simulink library "findDotPositions_ul"  (R2018b)
settings: Solver=VariableStepAuto  StartTime=0.0  StopTime=10.0  RelTol=1e-3
settings Model: Creator=MAE-NCSUCORE  LastModifiedBy=MAE-NCSUCORE

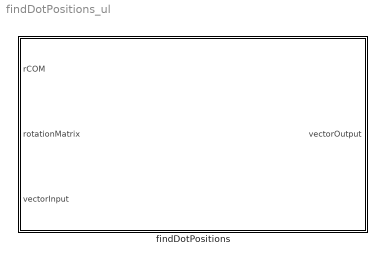
== system findDotPositions_ul ==
  findDotPositions : Subsystem

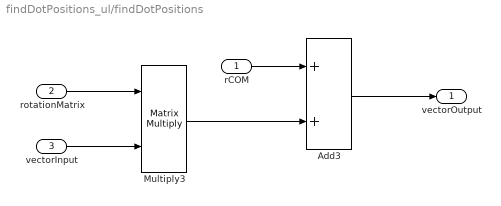
== system findDotPositions_ul/findDotPositions ==
  rCOM : Inport
  rotationMatrix : Inport  Port=2
  vectorInput : Inport  Port=3
  Add3 : Sum
  Multiply3 : Product  Multiplication=Matrix(*)
  vectorOutput : Outport
  wires:
  rCOM/1 -> Add3/1
  Multiply3/1 -> Add3/2
  vectorInput/1 -> Multiply3/2
  rotationMatrix/1 -> Multiply3/1
  Add3/1 -> vectorOutput/1
